simulink model "state_feedback"  (R2015a)
settings: Solver=ode45  StartTime=0.0  StopTime=10  RelTol=1e-6
values from neighbouring files (symbols this model uses):
  d0 = 1.5897e-3    (= 0.0015897)    [initialise.m]
  d1 = 1.773e-6    (= 1.773e-06)    [initialise.m]
  g = 9.81    [initialise.m]
  J0 = 1.4316e-4    (= 0.00014316)    [initialise.m]
  J1 = 2.078867e-4    (= 0.0002078867)    [initialise.m]
  K = lqi(sys_d,Q,R)    [BuildController.m]
  k = 350    [BuildController.m]
  Kf = 0.05722    [initialise.m]
  Kg = 13/18    (= 0.722222222222)    [initialise.m]
  Ki = K(5)    [BuildController.m]
  Kt = 0.05722    [initialise.m]
  L = place(sys_d.a',[1 0 0 0;0 0 1 0]',P)'    [BuildController.m]
  L0 = 0.09    [initialise.m]
  L1 = 0.225    [initialise.m]
  m1 = 0.009    [initialise.m]
  Ra = 17    [initialise.m]
undefined symbols (not defined in the file or in its folder): sigbuilder_block
undefined symbols (not defined in the file): n, sys_d
settings Model: Creator=Alvin  LastModifiedBy=Alvin
settings SolverCC: AlgebraicLoopSolver=LineSearch
settings DataIOCC: SaveState=on

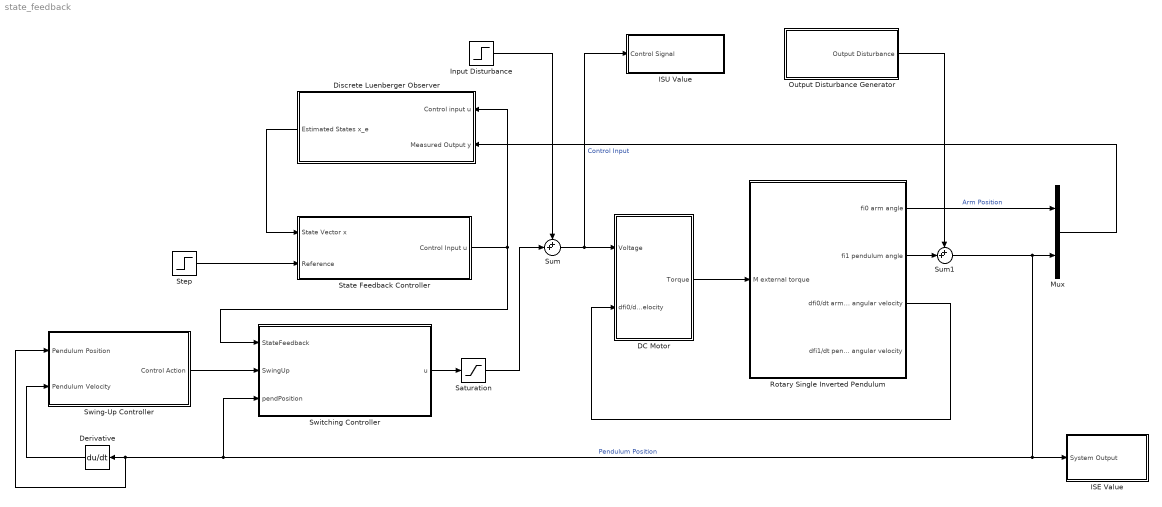
== system state_feedback ==
  DC Motor : Subsystem
  Derivative : Derivative
  Discrete Luenberger Observer : Subsystem  mask{A=sys_d.a, B=sys_d.b, C=[1 0 0 0; 0 0 1 0], L=L, SampleTime=0.025}
      mask prompts: A "Discretized state matrix A:"; B "Discretized input matrix B:"; C "Output matrix C:"; L "Discretized observer gain matrix L:"; SampleTime "Sample Time (-1 for inherited):"
      mask TypeOptions A: A/Gain
      mask TypeOptions B: B/Gain
      mask TypeOptions C: C/Gain
      mask TypeOptions L: L/Gain
      mask TypeOptions SampleTime:
      | Zero-Order
      | Hold1/SampleTime
      mask DialogControl DescTextVar Prompt: The Luenberger Observer block implements a discrete time Luenberger Observer. Use this block to estimate the states of an observable system using:  The discrete inputs and outputs of the system. A discrete state-space representation of the system. The Luenberger Observer is also sometimes referred to as a state observer or simply an observer.  You can control multi-input, multi-output systems by passing the output state vector of this block to a State Feedback Controller block.
  ISE Value : Subsystem
  ISU Value : Subsystem
  Input Disturbance : Step  Time=5  After=0  SampleTime=0
  Mux : Mux  Inputs=2
  Output Disturbance Generator : Subsystem  mask{Value=1}
      mask prompts: Value "Sinusoidal Disturbance (1) or Pulse Disturbance (0):"
      mask TypeOptions Value: Constant1/Value
      mask DialogControl DescTextVar Prompt: This block produces either a pulse output disturbnace or a sinusoidal disturbance. The disturbance is applied at t=5s of the simulation.
  Rotary Single Inverted Pendulum : Subsystem  mask{fi1=pi}
      mask prompts: fi1 "Pendulum Position Initial Condition"
      mask TypeOptions fi1: Pendulum/Constant/Value
  Saturation : Saturate  UpperLimit=12  LowerLimit=-12
  State Feedback Controller : Subsystem  mask{K=K(1:4), SampleTime=0.025}
      mask prompts: K "Feedback matrix K:"; SampleTime "Simulink:blkprm_prompts:AllBlksSampleTime"
      mask TypeOptions K: Gain/Gain
      mask TypeOptions SampleTime:
      | Zero-Order
      | Hold/SampleTime
      mask DialogControl DescTextVar Prompt: The State-Feedback Controller block implements a discrete-time state-feedback controller without integral action.
  Step : Step  Time=5  After=0  SampleTime=0
  Sum : Sum  Inputs=++|
  Sum1 : Sum  Inputs=++|
  Swing-Up Controller : Subsystem  mask{k=k, Upper=n*g, Lower=-n*g}
      mask prompts: k "Linear Swing-up gain k:"; Upper "Acceleration Saturation Constant n*g (Upper Limit):"; Lower "Acceleration Saturation Constant n*g (Lower Limit):"
      mask TypeOptions k: Gain/Gain
      mask TypeOptions Upper: Saturation1/UpperLimit
      mask TypeOptions Lower: Saturation1/LowerLimit
      mask DialogControl DescTextVar Prompt: Swing-up control action based on energy control techniques. The controller aims to change the energy of the system as fast as possible by ensuring the magnitude of the control action is as large as posssible.
  Switching Controller : MATLAB Function  TreatAsAtomicUnit=on
  wires:
  DC Motor/1(Torque) -> Rotary Single Inverted Pendulum/1(M external torque)
  Rotary Single Inverted Pendulum/3(dfi0/dt arm angular velocity) -> DC Motor/2(dfi0/dt Arm Angular Velocity)
  Step/1 -> State Feedback Controller/2(Reference)
  Rotary Single Inverted Pendulum/1(fi0 arm angle) -> Mux/1  "Arm Position"
  Discrete Luenberger Observer/1(Estimated States x_e) -> State Feedback Controller/1(State Vector x)
  Mux/1 -> Discrete Luenberger Observer/2(Measured Output y)
  State Feedback Controller/1(Control Input u) -> Switching Controller/1(StateFeedback), Discrete Luenberger Observer/1(Control input u)
  Switching Controller/1(u) -> Saturation/1
  Swing-Up Controller/1(Control Action) -> Switching Controller/2(SwingUp)
  Derivative/1 -> Swing-Up Controller/2(Pendulum Velocity)
  Sum/1 -> DC Motor/1(Voltage), ISU Value/1(Control Signal)  "Control Input"
  Saturation/1 -> Sum/2
  Input Disturbance/1 -> Sum/1
  Rotary Single Inverted Pendulum/2(fi1 pendulum angle) -> Sum1/2
  Sum1/1 -> Switching Controller/3(pendPosition), Swing-Up Controller/1(Pendulum Position), Derivative/1, ISE Value/1(System Output), Mux/2  "Pendulum Position"
  Output Disturbance Generator/1(Output Disturbance) -> Sum1/1

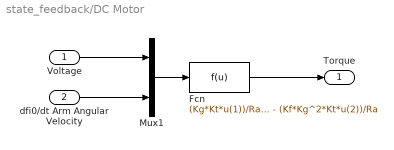
== system state_feedback/DC Motor ==
  Voltage : Inport
  dfi0/dt Arm Angular Velocity : Inport  Port=2
  Fcn : Fcn  Expr=(Kg*Kt*u(1))/Ra - (Kf*Kg^2*Kt*u(2))/Ra
  Mux1 : Mux  Inputs=2
  Torque : Outport
  wires:
  dfi0/dt Arm Angular Velocity/1 -> Mux1/2
  Mux1/1 -> Fcn/1
  Fcn/1 -> Torque/1
  Voltage/1 -> Mux1/1

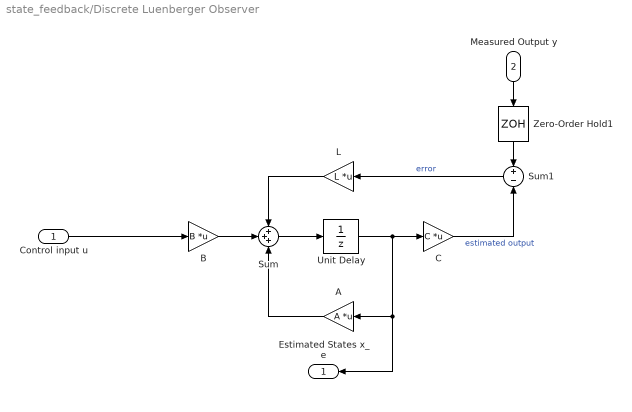
== system state_feedback/Discrete Luenberger Observer ==
  Control input u : Inport
  Measured Output y : Inport  Port=2
  A : Gain  Gain=A  Multiplication=Matrix(K*u)
  B : Gain  Gain=B  Multiplication=Matrix(K*u)
  C : Gain  Gain=C  Multiplication=Matrix(K*u)
  L : Gain  Gain=L  Multiplication=Matrix(K*u)
  Sum : Sum  Inputs=+++
  Sum1 : Sum  Inputs=+-
  Unit Delay : UnitDelay  SampleTime=-1
  Zero-Order Hold1 : ZeroOrderHold  SampleTime=SampleTime
  Estimated States x_e : Outport
  wires:
  Sum1/1 -> L/1  "error"
  A/1 -> Sum/3
  B/1 -> Sum/2
  C/1 -> Sum1/2  "estimated output"
  L/1 -> Sum/1
  Unit Delay/1 -> Estimated States x_e/1, A/1, C/1
  Sum/1 -> Unit Delay/1
  Control input u/1 -> B/1
  Measured Output y/1 -> Zero-Order Hold1/1
  Zero-Order Hold1/1 -> Sum1/1

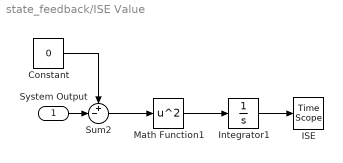
== system state_feedback/ISE Value ==
  System Output : Inport
  Constant : Constant  Value=0
  ISE : TimeScope
  Integrator1 : Integrator
  Math Function1 : Math  Operator=square  SaturateOnIntegerOverflow=on
  Sum2 : Sum  Inputs=+-|
  wires:
  Math Function1/1 -> Integrator1/1
  Constant/1 -> Sum2/1
  Sum2/1 -> Math Function1/1
  Integrator1/1 -> ISE/1
  System Output/1 -> Sum2/2

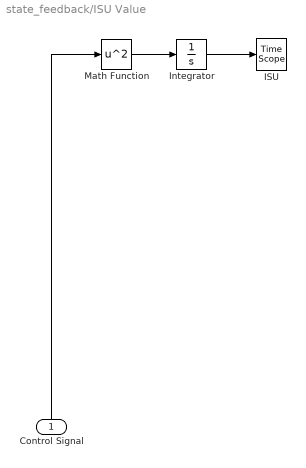
== system state_feedback/ISU Value ==
  Control Signal : Inport
  ISU : TimeScope
  Integrator : Integrator
  Math Function : Math  Operator=square  SaturateOnIntegerOverflow=on
  wires:
  Math Function/1 -> Integrator/1
  Integrator/1 -> ISU/1
  Control Signal/1 -> Math Function/1

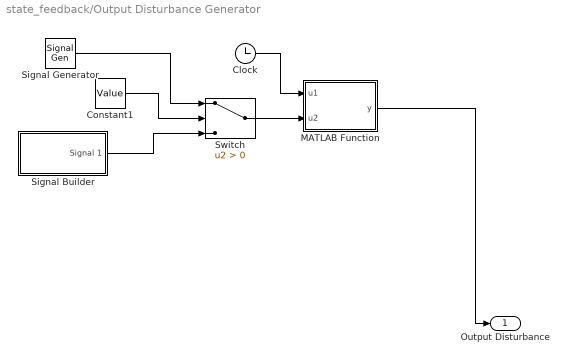
== system state_feedback/Output Disturbance Generator ==
  Clock : Clock
  Constant1 : Constant  Value=Value
  MATLAB Function : MATLAB Function  TreatAsAtomicUnit=on
  Signal Generator : SignalGenerator  Amplitude=0.05  Frequency=10  Units=rad/sec
  Signal Builder : Subsystem  Tag=STV Subsys  LoadFcn=sigbuilder_block('load');  StartFcn=sigbuilder_block('start');  StopFcn=sigbuilder_block('stop');  ClipboardFcn=sigbuilder_block('clipboard');  mask(Sigbuilder block){}
      mask help: Simulink:masks:SigbuilderBlock_MD
      mask init:
      | if ~strcmp(get_param(bdroot(gcbh),'SimulationStatus'),'stopped') tuvar = sigbuilder_block('maskInit'); end
      settings: CopyFcn=sigbuilder_block('copy');  DeleteFcn=sigbuilder_block('delete');  ModelCloseFcn=sigbuilder_block('modelClose');  PreSaveFcn=sigbuilder_block('preSave');  PauseFcn=sigbuilder_block('pause');  ContinueFcn=sigbuilder_block('continue');  NameChangeFcn=sigbuilder_block('namechange');  OpenFcn=sigbuilder_block('open',[437.6 199.2 550.4 400 ]);  CloseFcn=sigbuilder_block('close');
      mask Display: plot(0, 0, 100, 100,[2, 2, 32, 32, 2], [68, 8, 8, 68, 68],[32, 2], [38, 38], [32, 19, 2],[53, 60, 44], [32, 17, 17, 2],[16, 16, 31, 31]);txt = getActiveGroup(gcbh);text(2, 100, txt,'verticalAlignment', 'top');
  Switch : Switch  Criteria=u2 > Threshold
  Output Disturbance : Outport
  wires:
  Switch/1 -> MATLAB Function/2(u2)
  Clock/1 -> MATLAB Function/1(u1)
  MATLAB Function/1(y) -> Output Disturbance/1
  Signal Builder/1(Signal 1) -> Switch/3
  Signal Generator/1 -> Switch/1
  Constant1/1 -> Switch/2

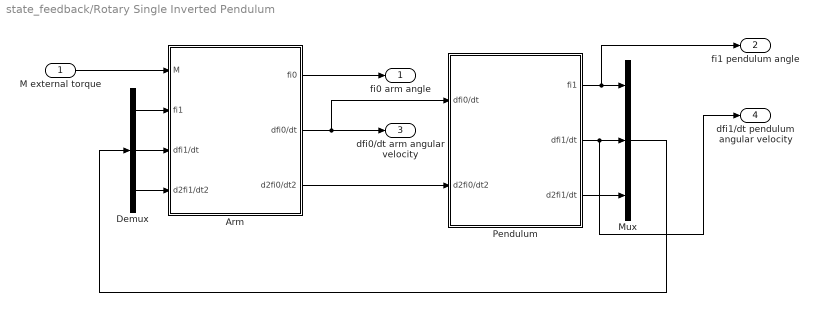
== system state_feedback/Rotary Single Inverted Pendulum ==
  M external torque : Inport
  Arm : Subsystem
  Demux : Demux  Outputs=3
  Mux : Mux  Inputs=3
  Pendulum : Subsystem
  fi0 arm angle : Outport
  fi1 pendulum angle : Outport  Port=2
  dfi0/dt arm angular velocity : Outport  Port=3
  dfi1/dt pendulum angular velocity : Outport  Port=4
  wires:
  Pendulum/1(fi1) -> fi1 pendulum angle/1, Mux/1
  Pendulum/2(dfi1/dt) -> dfi1/dt pendulum angular velocity/1, Mux/2
  Mux/1 -> Demux/1
  Demux/1 -> Arm/2(fi1)
  Demux/2 -> Arm/3(dfi1/dt)
  Demux/3 -> Arm/4(d2fi1/dt2)
  M external torque/1 -> Arm/1(M)
  Pendulum/3(d2fi1/dt) -> Mux/3
  Arm/3(d2fi0/dt2) -> Pendulum/2(d2fi0/dt2)
  Arm/1(fi0) -> fi0 arm angle/1
  Arm/2(dfi0/dt) -> dfi0/dt arm angular velocity/1, Pendulum/1(dfi0/dt)

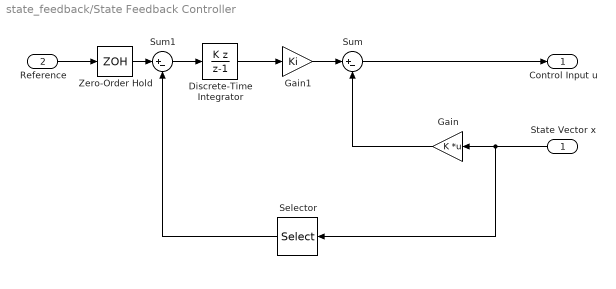
== system state_feedback/State Feedback Controller ==
  State Vector x : Inport
  Reference : Inport  Port=2
  Discrete-Time Integrator : DiscreteIntegrator  IntegratorMethod=Accumulation: Backward Euler  gainval=1  InitialConditionSetting=State (most efficient)  SampleTime=0.025
  Gain : Gain  Gain=K  Multiplication=Matrix(K*u)
  Gain1 : Gain  Gain=Ki
  Selector : Selector  InputPortWidth=4  Indices=[3]
  Sum : Sum  Inputs=|+-
  Sum1 : Sum  Inputs=|+-
  Zero-Order Hold : ZeroOrderHold  SampleTime=SampleTime
  Control Input u : Outport
  wires:
  Sum/1 -> Control Input u/1
  State Vector x/1 -> Selector/1, Gain/1
  Gain/1 -> Sum/2
  Reference/1 -> Zero-Order Hold/1
  Zero-Order Hold/1 -> Sum1/1
  Sum1/1 -> Discrete-Time Integrator/1
  Selector/1 -> Sum1/2
  Gain1/1 -> Sum/1
  Discrete-Time Integrator/1 -> Gain1/1

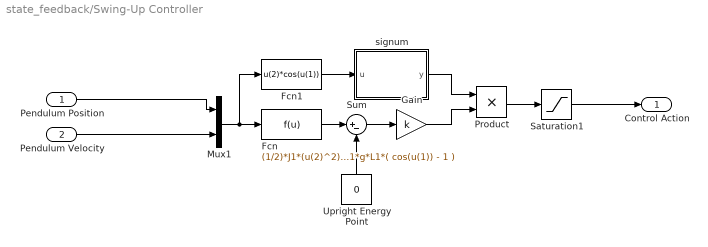
== system state_feedback/Swing-Up Controller ==
  Pendulum Position : Inport
  Pendulum Velocity : Inport  Port=2
  Fcn : Fcn  Expr=(1/2)*J1*(u(2)^2)+m1*g*L1*( cos(u(1)) - 1 )
  Fcn1 : Fcn  Expr=u(2)*cos(u(1))
  Gain : Gain  Gain=k
  Mux1 : Mux  Inputs=2
  Product : Product
  Saturation1 : Saturate  UpperLimit=Upper  LowerLimit=Lower
  Sum : Sum  Inputs=|+-
  Upright Energy Point : Constant  Value=0
  signum : MATLAB Function  TreatAsAtomicUnit=on
  Control Action : Outport
  wires:
  Product/1 -> Saturation1/1
  Upright Energy Point/1 -> Sum/2
  Mux1/1 -> Fcn1/1, Fcn/1
  Fcn/1 -> Sum/1
  Sum/1 -> Gain/1
  signum/1(y) -> Product/1
  Gain/1 -> Product/2
  Saturation1/1 -> Control Action/1
  Pendulum Velocity/1 -> Mux1/2
  Pendulum Position/1 -> Mux1/1
  Fcn1/1 -> signum/1(u)

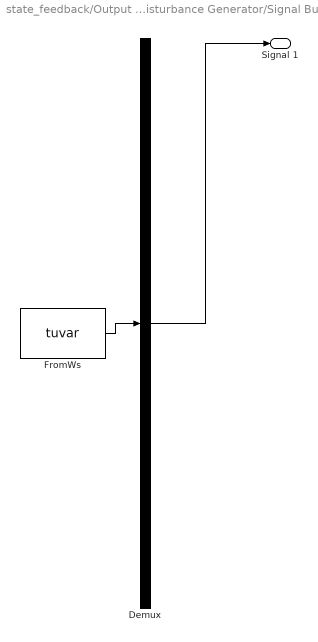
== system state_feedback/Output Disturbance Generator/Signal Builder ==
  Demux : Demux  Tag=STV Demux  Outputs=1
  FromWs : FromWorkspace  Tag=STV FromWs  VariableName=tuvar  SampleTime=0
      SigBuilderData=|
      | common.afterFinalStr = 'Extrapolate'
      | common.sampleTime = 0
      | dataSet.timeRange = [0 10]
      | dataSet.name = 'Group 1'
      | sbobj.Groups.Name = 'Group 1'
      | sbobj.Groups.Signals.Name = 'Signal 1'
      | sbobj.Groups.Signals.XData = [0 5 5 5.1 5.1 10]
      | sbobj.Groups.Signals.YData = [0 0 0.1 0.1 0 0]
  Signal 1 : Outport  Tag=STV Outport
  wires:
  Demux/1 -> Signal 1/1
  FromWs/1 -> Demux/1

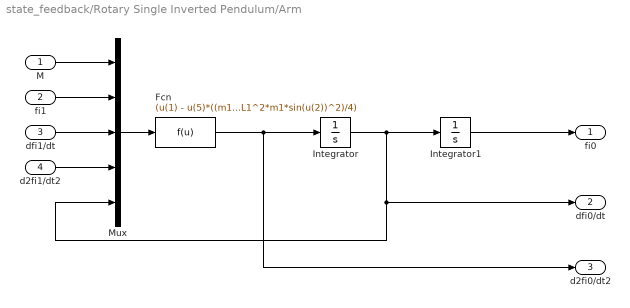
== system state_feedback/Rotary Single Inverted Pendulum/Arm ==
  M : Inport
  fi1 : Inport  Port=2
  dfi1/dt : Inport  Port=3
  d2fi1/dt2 : Inport  Port=4
  Fcn : Fcn  Expr=(u(1) - u(5)*((m1*u(3)*sin(2*u(2))*L1^2)/4 + d0) + (L0*L1*m1*u(3)^2*sin(u(2)))/2 - (L0*L1*m1*u(4)*cos(u(2)))/2)/(J0 + L0^2*m1 + (L1^2*m1*sin(u(2))^2)/4)
  Integrator : Integrator
  Integrator1 : Integrator
  Mux : Mux  Inputs=5
  fi0 : Outport
  dfi0/dt : Outport  Port=2
  d2fi0/dt2 : Outport  Port=3
  wires:
  Mux/1 -> Fcn/1
  Fcn/1 -> d2fi0/dt2/1, Integrator/1
  Integrator/1 -> dfi0/dt/1, Mux/5, Integrator1/1
  Integrator1/1 -> fi0/1
  fi1/1 -> Mux/2
  dfi1/dt/1 -> Mux/3
  M/1 -> Mux/1
  d2fi1/dt2/1 -> Mux/4

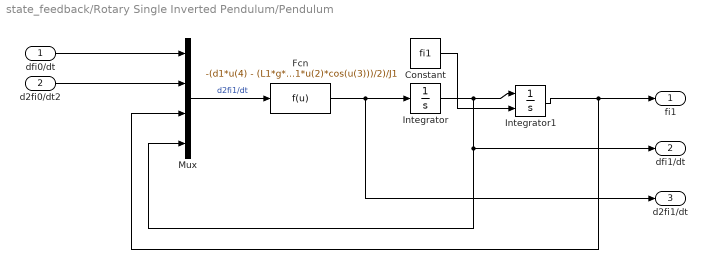
== system state_feedback/Rotary Single Inverted Pendulum/Pendulum ==
  dfi0/dt : Inport
  d2fi0/dt2 : Inport  Port=2
  Constant : Constant  Value=fi1
  Fcn : Fcn  Expr=-(d1*u(4) - (L1*g*m1*sin(u(3)))/2 - (L1^2*m1*u(1)^2*sin(2*u(3)))/8 + (L0*L1*m1*u(2)*cos(u(3)))/2)/J1
  Integrator : Integrator
  Integrator1 : Integrator  InitialConditionSource=external
  Mux : Mux
  fi1 : Outport
  dfi1/dt : Outport  Port=2
  d2fi1/dt : Outport  Port=3
  wires:
  Integrator1/1 -> fi1/1, Mux/3
  Fcn/1 -> d2fi1/dt/1, Integrator/1
  Mux/1 -> Fcn/1  "d2fi1/dt"
  Integrator/1 -> dfi1/dt/1, Mux/4, Integrator1/1
  dfi0/dt/1 -> Mux/1
  d2fi0/dt2/1 -> Mux/2
  Constant/1 -> Integrator1/2

== matlab function state_feedback/Switching Controller ==
  data: StateFeedback input; SwingUp input; u output; pendPosition input
function u  = switchControl(StateFeedback , SwingUp , pendPosition)

if (abs(pendPosition) <= 0.3)
    u = StateFeedback;
else
    u = SwingUp;
end

== matlab function state_feedback/Swing-Up Controller/signum ==
  data: u input; y output
function y = sgn(u)
%#codegen
if (u>= 0 )
    y = 1;
else
    y=-1;
end

== matlab function state_feedback/Output Disturbance Generator/MATLAB Function ==
  data: u1 input; y output; u2 input
function y = fcn(u1,u2)
%#codegen
if (u1>5)
    y = u2;
else
    y = 0;
end
